simulink model "nmsRR"  (R2021a)
settings: Solver=ode15s  StartTime=0.0  StopTime=t  MaxStep=1e-2  RelTol=1e-2
StartFcn:
  | tic
StopFcn:
  | toc
  | 
  | 
  | %if GimbalLockFlag
  |  % fprintf(2, 'Almost reached Gimbal Lock of IMU. Simulation stopped.\n')
  | %end
  | 
  | %fprintf('Elapsed time: %4.2f sec (%4.2f%% realtime)\n', a, tout(end)/a*100)
undefined symbols (not defined in the file): Balance02, Balance13, BalanceTrunk, BasisStim, CompensateSwing, CompliantLeg, FlexAnkle, Ground, ICs, init_des_left, init_des_right, init_l_left, init_l_right, init_q_del, init_sensor_body, init_sensor_world, init_v_left, init_v_right, LateralControl, mParams, PreventKneeOverextension, StepDur, Target02, Target13, theta0, X, Y, Z
libraries: simulink_extras x133, nesl_utility x105, sm_lib x88, simulink x72, robotcorelib x5, dspinverses x5, dspswit3 x2, vrlib x2, robotmaniplib x1
(part 6 of 8)

== system nmsRR/Spinal Layer/Stretch Reflex for Swing Leg Control/LPF 11x0.0025s ==
  in : Inport
  Demux2 : Demux  Outputs=11
  Mux2 : Mux  Inputs=11
  Transfer Fcn (with initial outputs)1 : simulink_extras/Additional Linear/Transfer Fcn (with initial outputs)  N=[1]  D="[0.0025  1]"  Y0=init_des_left(1)  U0=init_des_left(1)
  Transfer Fcn (with initial outputs)10 : simulink_extras/Additional Linear/Transfer Fcn (with initial outputs)  N=[1]  D="[0.0025  1]"  Y0=init_des_left(10)  U0=init_des_left(10)
  Transfer Fcn (with initial outputs)11 : simulink_extras/Additional Linear/Transfer Fcn (with initial outputs)  N=[1]  D="[0.0025  1]"  Y0=init_des_left(11)  U0=init_des_left(11)
  Transfer Fcn (with initial outputs)2 : simulink_extras/Additional Linear/Transfer Fcn (with initial outputs)  N=[1]  D="[0.0025  1]"  Y0=init_des_left(2)  U0=init_des_left(2)
  Transfer Fcn (with initial outputs)3 : simulink_extras/Additional Linear/Transfer Fcn (with initial outputs)  N=[1]  D="[0.0025  1]"  Y0=init_des_left(3)  U0=init_des_left(3)
  Transfer Fcn (with initial outputs)4 : simulink_extras/Additional Linear/Transfer Fcn (with initial outputs)  N=[1]  D="[0.0025  1]"  Y0=init_des_left(4)  U0=init_des_left(4)
  Transfer Fcn (with initial outputs)5 : simulink_extras/Additional Linear/Transfer Fcn (with initial outputs)  N=[1]  D="[0.0025  1]"  Y0=init_des_left(5)  U0=init_des_left(5)
  Transfer Fcn (with initial outputs)6 : simulink_extras/Additional Linear/Transfer Fcn (with initial outputs)  N=[1]  D="[0.0025  1]"  Y0=init_des_left(6)  U0=init_des_left(6)
  Transfer Fcn (with initial outputs)7 : simulink_extras/Additional Linear/Transfer Fcn (with initial outputs)  N=[1]  D="[0.0025  1]"  Y0=init_des_left(7)  U0=init_des_left(7)
  Transfer Fcn (with initial outputs)8 : simulink_extras/Additional Linear/Transfer Fcn (with initial outputs)  N=[1]  D="[0.0025  1]"  Y0=init_des_left(8)  U0=init_des_left(8)
  Transfer Fcn (with initial outputs)9 : simulink_extras/Additional Linear/Transfer Fcn (with initial outputs)  N=[1]  D="[0.0025  1]"  Y0=init_des_left(9)  U0=init_des_left(9)
  lambda : Outport
  wires:
  Mux2/1 -> lambda/1
  Demux2/1 -> Transfer Fcn (with initial outputs)1/1
  Transfer Fcn (with initial outputs)6/1 -> Mux2/6
  Transfer Fcn (with initial outputs)3/1 -> Mux2/3
  Transfer Fcn (with initial outputs)10/1 -> Mux2/10
  Demux2/2 -> Transfer Fcn (with initial outputs)2/1
  Transfer Fcn (with initial outputs)7/1 -> Mux2/7
  Demux2/10 -> Transfer Fcn (with initial outputs)10/1
  Transfer Fcn (with initial outputs)9/1 -> Mux2/9
  Demux2/9 -> Transfer Fcn (with initial outputs)9/1
  in/1 -> Demux2/1
  Transfer Fcn (with initial outputs)4/1 -> Mux2/4
  Transfer Fcn (with initial outputs)8/1 -> Mux2/8
  Transfer Fcn (with initial outputs)5/1 -> Mux2/5
  Transfer Fcn (with initial outputs)11/1 -> Mux2/11
  Demux2/11 -> Transfer Fcn (with initial outputs)11/1
  Demux2/7 -> Transfer Fcn (with initial outputs)7/1
  Demux2/3 -> Transfer Fcn (with initial outputs)3/1
  Demux2/6 -> Transfer Fcn (with initial outputs)6/1
  Transfer Fcn (with initial outputs)1/1 -> Mux2/1
  Demux2/5 -> Transfer Fcn (with initial outputs)5/1
  Transfer Fcn (with initial outputs)2/1 -> Mux2/2
  Demux2/4 -> Transfer Fcn (with initial outputs)4/1
  Demux2/8 -> Transfer Fcn (with initial outputs)8/1

== system nmsRR/Spinal Layer/Stretch Reflex for Swing Leg Control/LPF 11x0.0025s1 ==
  in : Inport
  Demux2 : Demux  Outputs=11
  Mux2 : Mux  Inputs=11
  Transfer Fcn (with initial outputs)1 : simulink_extras/Additional Linear/Transfer Fcn (with initial outputs)  N=[1]  D="[0.0025  1]"  Y0=init_l_left(1)  U0=init_l_left(1)
  Transfer Fcn (with initial outputs)10 : simulink_extras/Additional Linear/Transfer Fcn (with initial outputs)  N=[1]  D="[0.0025  1]"  Y0=init_l_left(10)  U0=init_l_left(10)
  Transfer Fcn (with initial outputs)11 : simulink_extras/Additional Linear/Transfer Fcn (with initial outputs)  N=[1]  D="[0.0025  1]"  Y0=init_l_left(11)  U0=init_l_left(11)
  Transfer Fcn (with initial outputs)2 : simulink_extras/Additional Linear/Transfer Fcn (with initial outputs)  N=[1]  D="[0.0025  1]"  Y0=init_l_left(2)  U0=init_l_left(2)
  Transfer Fcn (with initial outputs)3 : simulink_extras/Additional Linear/Transfer Fcn (with initial outputs)  N=[1]  D="[0.0025  1]"  Y0=init_l_left(3)  U0=init_l_left(3)
  Transfer Fcn (with initial outputs)4 : simulink_extras/Additional Linear/Transfer Fcn (with initial outputs)  N=[1]  D="[0.0025  1]"  Y0=init_l_left(4)  U0=init_l_left(4)
  Transfer Fcn (with initial outputs)5 : simulink_extras/Additional Linear/Transfer Fcn (with initial outputs)  N=[1]  D="[0.0025  1]"  Y0=init_l_left(5)  U0=init_l_left(5)
  Transfer Fcn (with initial outputs)6 : simulink_extras/Additional Linear/Transfer Fcn (with initial outputs)  N=[1]  D="[0.0025  1]"  Y0=init_l_left(6)  U0=init_l_left(6)
  Transfer Fcn (with initial outputs)7 : simulink_extras/Additional Linear/Transfer Fcn (with initial outputs)  N=[1]  D="[0.0025  1]"  Y0=init_l_left(7)  U0=init_l_left(7)
  Transfer Fcn (with initial outputs)8 : simulink_extras/Additional Linear/Transfer Fcn (with initial outputs)  N=[1]  D="[0.0025  1]"  Y0=init_l_left(8)  U0=init_l_left(8)
  Transfer Fcn (with initial outputs)9 : simulink_extras/Additional Linear/Transfer Fcn (with initial outputs)  N=[1]  D="[0.0025  1]"  Y0=init_l_left(9)  U0=init_l_left(9)
  l : Outport
  wires:
  Mux2/1 -> l/1
  Demux2/1 -> Transfer Fcn (with initial outputs)1/1
  Transfer Fcn (with initial outputs)6/1 -> Mux2/6
  Transfer Fcn (with initial outputs)3/1 -> Mux2/3
  Transfer Fcn (with initial outputs)10/1 -> Mux2/10
  Demux2/2 -> Transfer Fcn (with initial outputs)2/1
  Transfer Fcn (with initial outputs)7/1 -> Mux2/7
  Demux2/10 -> Transfer Fcn (with initial outputs)10/1
  Transfer Fcn (with initial outputs)9/1 -> Mux2/9
  Demux2/9 -> Transfer Fcn (with initial outputs)9/1
  in/1 -> Demux2/1
  Transfer Fcn (with initial outputs)4/1 -> Mux2/4
  Transfer Fcn (with initial outputs)8/1 -> Mux2/8
  Transfer Fcn (with initial outputs)5/1 -> Mux2/5
  Transfer Fcn (with initial outputs)11/1 -> Mux2/11
  Demux2/11 -> Transfer Fcn (with initial outputs)11/1
  Demux2/7 -> Transfer Fcn (with initial outputs)7/1
  Demux2/3 -> Transfer Fcn (with initial outputs)3/1
  Demux2/6 -> Transfer Fcn (with initial outputs)6/1
  Transfer Fcn (with initial outputs)1/1 -> Mux2/1
  Demux2/5 -> Transfer Fcn (with initial outputs)5/1
  Transfer Fcn (with initial outputs)2/1 -> Mux2/2
  Demux2/4 -> Transfer Fcn (with initial outputs)4/1
  Demux2/8 -> Transfer Fcn (with initial outputs)8/1

== system nmsRR/Spinal Layer/Stretch Reflex for Swing Leg Control/LPF 11x0.0025s2 ==
  in : Inport
  Demux2 : Demux  Outputs=11
  Mux2 : Mux  Inputs=11
  Transfer Fcn (with initial outputs)1 : simulink_extras/Additional Linear/Transfer Fcn (with initial outputs)  N=[1]  D="[0.0025  1]"  Y0=init_v_left(1)  U0=init_v_left(1)
  Transfer Fcn (with initial outputs)10 : simulink_extras/Additional Linear/Transfer Fcn (with initial outputs)  N=[1]  D="[0.0025  1]"  Y0=init_v_left(10)  U0=init_v_left(10)
  Transfer Fcn (with initial outputs)11 : simulink_extras/Additional Linear/Transfer Fcn (with initial outputs)  N=[1]  D="[0.0025  1]"  Y0=init_v_left(11)  U0=init_v_left(11)
  Transfer Fcn (with initial outputs)2 : simulink_extras/Additional Linear/Transfer Fcn (with initial outputs)  N=[1]  D="[0.0025  1]"  Y0=init_v_left(2)  U0=init_v_left(2)
  Transfer Fcn (with initial outputs)3 : simulink_extras/Additional Linear/Transfer Fcn (with initial outputs)  N=[1]  D="[0.0025  1]"  Y0=init_v_left(3)  U0=init_v_left(3)
  Transfer Fcn (with initial outputs)4 : simulink_extras/Additional Linear/Transfer Fcn (with initial outputs)  N=[1]  D="[0.0025  1]"  Y0=init_v_left(4)  U0=init_v_left(4)
  Transfer Fcn (with initial outputs)5 : simulink_extras/Additional Linear/Transfer Fcn (with initial outputs)  N=[1]  D="[0.0025  1]"  Y0=init_v_left(5)  U0=init_v_left(5)
  Transfer Fcn (with initial outputs)6 : simulink_extras/Additional Linear/Transfer Fcn (with initial outputs)  N=[1]  D="[0.0025  1]"  Y0=init_v_left(6)  U0=init_v_left(6)
  Transfer Fcn (with initial outputs)7 : simulink_extras/Additional Linear/Transfer Fcn (with initial outputs)  N=[1]  D="[0.0025  1]"  Y0=init_v_left(7)  U0=init_v_left(7)
  Transfer Fcn (with initial outputs)8 : simulink_extras/Additional Linear/Transfer Fcn (with initial outputs)  N=[1]  D="[0.0025  1]"  Y0=init_v_left(8)  U0=init_v_left(8)
  Transfer Fcn (with initial outputs)9 : simulink_extras/Additional Linear/Transfer Fcn (with initial outputs)  N=[1]  D="[0.0025  1]"  Y0=init_v_left(9)  U0=init_v_left(9)
  v : Outport
  wires:
  Mux2/1 -> v/1
  Demux2/1 -> Transfer Fcn (with initial outputs)1/1
  Transfer Fcn (with initial outputs)6/1 -> Mux2/6
  Transfer Fcn (with initial outputs)3/1 -> Mux2/3
  Transfer Fcn (with initial outputs)10/1 -> Mux2/10
  Demux2/2 -> Transfer Fcn (with initial outputs)2/1
  Transfer Fcn (with initial outputs)7/1 -> Mux2/7
  Demux2/10 -> Transfer Fcn (with initial outputs)10/1
  Transfer Fcn (with initial outputs)9/1 -> Mux2/9
  Demux2/9 -> Transfer Fcn (with initial outputs)9/1
  in/1 -> Demux2/1
  Transfer Fcn (with initial outputs)4/1 -> Mux2/4
  Transfer Fcn (with initial outputs)8/1 -> Mux2/8
  Transfer Fcn (with initial outputs)5/1 -> Mux2/5
  Transfer Fcn (with initial outputs)11/1 -> Mux2/11
  Demux2/11 -> Transfer Fcn (with initial outputs)11/1
  Demux2/7 -> Transfer Fcn (with initial outputs)7/1
  Demux2/3 -> Transfer Fcn (with initial outputs)3/1
  Demux2/6 -> Transfer Fcn (with initial outputs)6/1
  Transfer Fcn (with initial outputs)1/1 -> Mux2/1
  Demux2/5 -> Transfer Fcn (with initial outputs)5/1
  Transfer Fcn (with initial outputs)2/1 -> Mux2/2
  Demux2/4 -> Transfer Fcn (with initial outputs)4/1
  Demux2/8 -> Transfer Fcn (with initial outputs)8/1

== system nmsRR/Spinal Layer/Stretch Reflex for Swing Leg Control/LPF 11x0.0025s3 ==
  in : Inport
  Demux2 : Demux  Outputs=11
  Mux2 : Mux  Inputs=11
  Transfer Fcn (with initial outputs)1 : simulink_extras/Additional Linear/Transfer Fcn (with initial outputs)  N=[1]  D="[0.0025  1]"  Y0=init_des_right(1)  U0=init_des_right(1)
  Transfer Fcn (with initial outputs)10 : simulink_extras/Additional Linear/Transfer Fcn (with initial outputs)  N=[1]  D="[0.0025  1]"  Y0=init_des_right(10)  U0=init_des_right(10)
  Transfer Fcn (with initial outputs)11 : simulink_extras/Additional Linear/Transfer Fcn (with initial outputs)  N=[1]  D="[0.0025  1]"  Y0=init_des_right(11)  U0=init_des_right(11)
  Transfer Fcn (with initial outputs)2 : simulink_extras/Additional Linear/Transfer Fcn (with initial outputs)  N=[1]  D="[0.0025  1]"  Y0=init_des_right(2)  U0=init_des_right(2)
  Transfer Fcn (with initial outputs)3 : simulink_extras/Additional Linear/Transfer Fcn (with initial outputs)  N=[1]  D="[0.0025  1]"  Y0=init_des_right(3)  U0=init_des_right(3)
  Transfer Fcn (with initial outputs)4 : simulink_extras/Additional Linear/Transfer Fcn (with initial outputs)  N=[1]  D="[0.0025  1]"  Y0=init_des_right(4)  U0=init_des_right(4)
  Transfer Fcn (with initial outputs)5 : simulink_extras/Additional Linear/Transfer Fcn (with initial outputs)  N=[1]  D="[0.0025  1]"  Y0=init_des_right(5)  U0=init_des_right(5)
  Transfer Fcn (with initial outputs)6 : simulink_extras/Additional Linear/Transfer Fcn (with initial outputs)  N=[1]  D="[0.0025  1]"  Y0=init_des_right(6)  U0=init_des_right(6)
  Transfer Fcn (with initial outputs)7 : simulink_extras/Additional Linear/Transfer Fcn (with initial outputs)  N=[1]  D="[0.0025  1]"  Y0=init_des_right(7)  U0=init_des_right(7)
  Transfer Fcn (with initial outputs)8 : simulink_extras/Additional Linear/Transfer Fcn (with initial outputs)  N=[1]  D="[0.0025  1]"  Y0=init_des_right(8)  U0=init_des_right(8)
  Transfer Fcn (with initial outputs)9 : simulink_extras/Additional Linear/Transfer Fcn (with initial outputs)  N=[1]  D="[0.0025  1]"  Y0=init_des_right(9)  U0=init_des_right(9)
  lambda : Outport
  wires:
  Mux2/1 -> lambda/1
  Demux2/1 -> Transfer Fcn (with initial outputs)1/1
  Transfer Fcn (with initial outputs)6/1 -> Mux2/6
  Transfer Fcn (with initial outputs)3/1 -> Mux2/3
  Transfer Fcn (with initial outputs)10/1 -> Mux2/10
  Demux2/2 -> Transfer Fcn (with initial outputs)2/1
  Transfer Fcn (with initial outputs)7/1 -> Mux2/7
  Demux2/10 -> Transfer Fcn (with initial outputs)10/1
  Transfer Fcn (with initial outputs)9/1 -> Mux2/9
  Demux2/9 -> Transfer Fcn (with initial outputs)9/1
  in/1 -> Demux2/1
  Transfer Fcn (with initial outputs)4/1 -> Mux2/4
  Transfer Fcn (with initial outputs)8/1 -> Mux2/8
  Transfer Fcn (with initial outputs)5/1 -> Mux2/5
  Transfer Fcn (with initial outputs)11/1 -> Mux2/11
  Demux2/11 -> Transfer Fcn (with initial outputs)11/1
  Demux2/7 -> Transfer Fcn (with initial outputs)7/1
  Demux2/3 -> Transfer Fcn (with initial outputs)3/1
  Demux2/6 -> Transfer Fcn (with initial outputs)6/1
  Transfer Fcn (with initial outputs)1/1 -> Mux2/1
  Demux2/5 -> Transfer Fcn (with initial outputs)5/1
  Transfer Fcn (with initial outputs)2/1 -> Mux2/2
  Demux2/4 -> Transfer Fcn (with initial outputs)4/1
  Demux2/8 -> Transfer Fcn (with initial outputs)8/1

== system nmsRR/Spinal Layer/Stretch Reflex for Swing Leg Control/LPF 11x0.0025s4 ==
  in : Inport
  Demux2 : Demux  Outputs=11
  Mux2 : Mux  Inputs=11
  Transfer Fcn (with initial outputs)1 : simulink_extras/Additional Linear/Transfer Fcn (with initial outputs)  N=[1]  D="[0.0025  1]"  Y0=init_l_right(1)  U0=init_l_right(1)
  Transfer Fcn (with initial outputs)10 : simulink_extras/Additional Linear/Transfer Fcn (with initial outputs)  N=[1]  D="[0.0025  1]"  Y0=init_l_right(10)  U0=init_l_right(10)
  Transfer Fcn (with initial outputs)11 : simulink_extras/Additional Linear/Transfer Fcn (with initial outputs)  N=[1]  D="[0.0025  1]"  Y0=init_l_right(11)  U0=init_l_right(11)
  Transfer Fcn (with initial outputs)2 : simulink_extras/Additional Linear/Transfer Fcn (with initial outputs)  N=[1]  D="[0.0025  1]"  Y0=init_l_right(2)  U0=init_l_right(2)
  Transfer Fcn (with initial outputs)3 : simulink_extras/Additional Linear/Transfer Fcn (with initial outputs)  N=[1]  D="[0.0025  1]"  Y0=init_l_right(3)  U0=init_l_right(3)
  Transfer Fcn (with initial outputs)4 : simulink_extras/Additional Linear/Transfer Fcn (with initial outputs)  N=[1]  D="[0.0025  1]"  Y0=init_l_right(4)  U0=init_l_right(4)
  Transfer Fcn (with initial outputs)5 : simulink_extras/Additional Linear/Transfer Fcn (with initial outputs)  N=[1]  D="[0.0025  1]"  Y0=init_l_right(5)  U0=init_l_right(5)
  Transfer Fcn (with initial outputs)6 : simulink_extras/Additional Linear/Transfer Fcn (with initial outputs)  N=[1]  D="[0.0025  1]"  Y0=init_l_right(6)  U0=init_l_right(6)
  Transfer Fcn (with initial outputs)7 : simulink_extras/Additional Linear/Transfer Fcn (with initial outputs)  N=[1]  D="[0.0025  1]"  Y0=init_l_right(7)  U0=init_l_right(7)
  Transfer Fcn (with initial outputs)8 : simulink_extras/Additional Linear/Transfer Fcn (with initial outputs)  N=[1]  D="[0.0025  1]"  Y0=init_l_right(8)  U0=init_l_right(8)
  Transfer Fcn (with initial outputs)9 : simulink_extras/Additional Linear/Transfer Fcn (with initial outputs)  N=[1]  D="[0.0025  1]"  Y0=init_l_right(9)  U0=init_l_right(9)
  l : Outport
  wires:
  Mux2/1 -> l/1
  Demux2/1 -> Transfer Fcn (with initial outputs)1/1
  Transfer Fcn (with initial outputs)6/1 -> Mux2/6
  Transfer Fcn (with initial outputs)3/1 -> Mux2/3
  Transfer Fcn (with initial outputs)10/1 -> Mux2/10
  Demux2/2 -> Transfer Fcn (with initial outputs)2/1
  Transfer Fcn (with initial outputs)7/1 -> Mux2/7
  Demux2/10 -> Transfer Fcn (with initial outputs)10/1
  Transfer Fcn (with initial outputs)9/1 -> Mux2/9
  Demux2/9 -> Transfer Fcn (with initial outputs)9/1
  in/1 -> Demux2/1
  Transfer Fcn (with initial outputs)4/1 -> Mux2/4
  Transfer Fcn (with initial outputs)8/1 -> Mux2/8
  Transfer Fcn (with initial outputs)5/1 -> Mux2/5
  Transfer Fcn (with initial outputs)11/1 -> Mux2/11
  Demux2/11 -> Transfer Fcn (with initial outputs)11/1
  Demux2/7 -> Transfer Fcn (with initial outputs)7/1
  Demux2/3 -> Transfer Fcn (with initial outputs)3/1
  Demux2/6 -> Transfer Fcn (with initial outputs)6/1
  Transfer Fcn (with initial outputs)1/1 -> Mux2/1
  Demux2/5 -> Transfer Fcn (with initial outputs)5/1
  Transfer Fcn (with initial outputs)2/1 -> Mux2/2
  Demux2/4 -> Transfer Fcn (with initial outputs)4/1
  Demux2/8 -> Transfer Fcn (with initial outputs)8/1

== system nmsRR/Spinal Layer/Stretch Reflex for Swing Leg Control/LPF 11x0.0025s5 ==
  in : Inport
  Demux2 : Demux  Outputs=11
  Mux2 : Mux  Inputs=11
  Transfer Fcn (with initial outputs){1..11} (11 alike) : simulink_extras/Additional Linear/Transfer Fcn (with initial outputs)  N=[ 1 0]  D="[0.0025  1]"  Y0=0  U0=0
  lambda dot : Outport
  wires:
  Mux2/1 -> lambda dot/1
  Demux2/1 -> Transfer Fcn (with initial outputs)1/1
  Transfer Fcn (with initial outputs)6/1 -> Mux2/6
  Transfer Fcn (with initial outputs)3/1 -> Mux2/3
  Transfer Fcn (with initial outputs)10/1 -> Mux2/10
  Demux2/2 -> Transfer Fcn (with initial outputs)2/1
  Transfer Fcn (with initial outputs)7/1 -> Mux2/7
  Demux2/10 -> Transfer Fcn (with initial outputs)10/1
  Transfer Fcn (with initial outputs)9/1 -> Mux2/9
  Demux2/9 -> Transfer Fcn (with initial outputs)9/1
  in/1 -> Demux2/1
  Transfer Fcn (with initial outputs)4/1 -> Mux2/4
  Transfer Fcn (with initial outputs)8/1 -> Mux2/8
  Transfer Fcn (with initial outputs)5/1 -> Mux2/5
  Transfer Fcn (with initial outputs)11/1 -> Mux2/11
  Demux2/11 -> Transfer Fcn (with initial outputs)11/1
  Demux2/7 -> Transfer Fcn (with initial outputs)7/1
  Demux2/3 -> Transfer Fcn (with initial outputs)3/1
  Demux2/6 -> Transfer Fcn (with initial outputs)6/1
  Transfer Fcn (with initial outputs)1/1 -> Mux2/1
  Demux2/5 -> Transfer Fcn (with initial outputs)5/1
  Transfer Fcn (with initial outputs)2/1 -> Mux2/2
  Demux2/4 -> Transfer Fcn (with initial outputs)4/1
  Demux2/8 -> Transfer Fcn (with initial outputs)8/1

== system nmsRR/Spinal Layer/Stretch Reflex for Swing Leg Control/LPF 11x0.0025s6 ==
  in : Inport
  Demux2 : Demux  Outputs=11
  Mux2 : Mux  Inputs=11
  Transfer Fcn (with initial outputs)1 : simulink_extras/Additional Linear/Transfer Fcn (with initial outputs)  N=[1]  D="[0.0025  1]"  Y0=init_v_right(1)  U0=init_v_right(1)
  Transfer Fcn (with initial outputs)10 : simulink_extras/Additional Linear/Transfer Fcn (with initial outputs)  N=[1]  D="[0.0025  1]"  Y0=init_v_right(10)  U0=init_v_right(10)
  Transfer Fcn (with initial outputs)11 : simulink_extras/Additional Linear/Transfer Fcn (with initial outputs)  N=[1]  D="[0.0025  1]"  Y0=init_v_right(11)  U0=init_v_right(11)
  Transfer Fcn (with initial outputs)2 : simulink_extras/Additional Linear/Transfer Fcn (with initial outputs)  N=[1]  D="[0.0025  1]"  Y0=init_v_right(2)  U0=init_v_right(2)
  Transfer Fcn (with initial outputs)3 : simulink_extras/Additional Linear/Transfer Fcn (with initial outputs)  N=[1]  D="[0.0025  1]"  Y0=init_v_right(3)  U0=init_v_right(3)
  Transfer Fcn (with initial outputs)4 : simulink_extras/Additional Linear/Transfer Fcn (with initial outputs)  N=[1]  D="[0.0025  1]"  Y0=init_v_right(4)  U0=init_v_right(4)
  Transfer Fcn (with initial outputs)5 : simulink_extras/Additional Linear/Transfer Fcn (with initial outputs)  N=[1]  D="[0.0025  1]"  Y0=init_v_right(5)  U0=init_v_right(5)
  Transfer Fcn (with initial outputs)6 : simulink_extras/Additional Linear/Transfer Fcn (with initial outputs)  N=[1]  D="[0.0025  1]"  Y0=init_v_right(6)  U0=init_v_right(6)
  Transfer Fcn (with initial outputs)7 : simulink_extras/Additional Linear/Transfer Fcn (with initial outputs)  N=[1]  D="[0.0025  1]"  Y0=init_v_right(7)  U0=init_v_right(7)
  Transfer Fcn (with initial outputs)8 : simulink_extras/Additional Linear/Transfer Fcn (with initial outputs)  N=[1]  D="[0.0025  1]"  Y0=init_v_right(8)  U0=init_v_right(8)
  Transfer Fcn (with initial outputs)9 : simulink_extras/Additional Linear/Transfer Fcn (with initial outputs)  N=[1]  D="[0.0025  1]"  Y0=init_v_right(9)  U0=init_v_right(9)
  v : Outport
  wires:
  Mux2/1 -> v/1
  Demux2/1 -> Transfer Fcn (with initial outputs)1/1
  Transfer Fcn (with initial outputs)6/1 -> Mux2/6
  Transfer Fcn (with initial outputs)3/1 -> Mux2/3
  Transfer Fcn (with initial outputs)10/1 -> Mux2/10
  Demux2/2 -> Transfer Fcn (with initial outputs)2/1
  Transfer Fcn (with initial outputs)7/1 -> Mux2/7
  Demux2/10 -> Transfer Fcn (with initial outputs)10/1
  Transfer Fcn (with initial outputs)9/1 -> Mux2/9
  Demux2/9 -> Transfer Fcn (with initial outputs)9/1
  in/1 -> Demux2/1
  Transfer Fcn (with initial outputs)4/1 -> Mux2/4
  Transfer Fcn (with initial outputs)8/1 -> Mux2/8
  Transfer Fcn (with initial outputs)5/1 -> Mux2/5
  Transfer Fcn (with initial outputs)11/1 -> Mux2/11
  Demux2/11 -> Transfer Fcn (with initial outputs)11/1
  Demux2/7 -> Transfer Fcn (with initial outputs)7/1
  Demux2/3 -> Transfer Fcn (with initial outputs)3/1
  Demux2/6 -> Transfer Fcn (with initial outputs)6/1
  Transfer Fcn (with initial outputs)1/1 -> Mux2/1
  Demux2/5 -> Transfer Fcn (with initial outputs)5/1
  Transfer Fcn (with initial outputs)2/1 -> Mux2/2
  Demux2/4 -> Transfer Fcn (with initial outputs)4/1
  Demux2/8 -> Transfer Fcn (with initial outputs)8/1

== system nmsRR/Spinal Layer/Stretch Reflex for Swing Leg Control/LPF 11x0.0025s7 ==
  in : Inport
  Demux2 : Demux  Outputs=11
  Mux2 : Mux  Inputs=11
  Transfer Fcn (with initial outputs){1..11} (11 alike) : simulink_extras/Additional Linear/Transfer Fcn (with initial outputs)  N=[ 1 0]  D="[0.0025  1]"  Y0=0  U0=0
  lambda dot : Outport
  wires:
  Mux2/1 -> lambda dot/1
  Demux2/1 -> Transfer Fcn (with initial outputs)1/1
  Transfer Fcn (with initial outputs)6/1 -> Mux2/6
  Transfer Fcn (with initial outputs)3/1 -> Mux2/3
  Transfer Fcn (with initial outputs)10/1 -> Mux2/10
  Demux2/2 -> Transfer Fcn (with initial outputs)2/1
  Transfer Fcn (with initial outputs)7/1 -> Mux2/7
  Demux2/10 -> Transfer Fcn (with initial outputs)10/1
  Transfer Fcn (with initial outputs)9/1 -> Mux2/9
  Demux2/9 -> Transfer Fcn (with initial outputs)9/1
  in/1 -> Demux2/1
  Transfer Fcn (with initial outputs)4/1 -> Mux2/4
  Transfer Fcn (with initial outputs)8/1 -> Mux2/8
  Transfer Fcn (with initial outputs)5/1 -> Mux2/5
  Transfer Fcn (with initial outputs)11/1 -> Mux2/11
  Demux2/11 -> Transfer Fcn (with initial outputs)11/1
  Demux2/7 -> Transfer Fcn (with initial outputs)7/1
  Demux2/3 -> Transfer Fcn (with initial outputs)3/1
  Demux2/6 -> Transfer Fcn (with initial outputs)6/1
  Transfer Fcn (with initial outputs)1/1 -> Mux2/1
  Demux2/5 -> Transfer Fcn (with initial outputs)5/1
  Transfer Fcn (with initial outputs)2/1 -> Mux2/2
  Demux2/4 -> Transfer Fcn (with initial outputs)4/1
  Demux2/8 -> Transfer Fcn (with initial outputs)8/1

== system nmsRR/Spinal Layer/Stretch Reflex for Swing Leg Control/Stretch Reflex Left ==
  lambda : Inport
  lambda_dot : Inport  Port=2
  l_ce : Inport  Port=3
  v_ce : Inport  Port=4
  Add2 : Sum  Inputs=-+
  Add3 : Sum  Inputs=-+
  Add7 : Sum
  Gain10 : Gain  Gain=0.03
  Gain9 : Gain  Gain=mParams.muscles.K
  STIM : Outport  VectorParamsAs1DForOutWhenUnconnected=off
  wires:
  lambda/1 -> Add2/1
  Add7/1 -> STIM/1
  Gain9/1 -> Add7/1
  Gain10/1 -> Add7/2
  Add3/1 -> Gain10/1
  Add2/1 -> Gain9/1
  v_ce/1 -> Add3/2
  l_ce/1 -> Add2/2
  lambda_dot/1 -> Add3/1

== system nmsRR/Spinal Layer/Stretch Reflex for Swing Leg Control/Stretch Reflex Right ==
  lambda : Inport
  lambda_dot : Inport  Port=2
  l_ce : Inport  Port=3
  v_ce : Inport  Port=4
  Add2 : Sum  Inputs=-+
  Add3 : Sum  Inputs=-+
  Add7 : Sum
  Gain1 : Gain  Commented=on  Gain=[ 0.03 0.03 0.03 0.03 0.03 0.03 0.03 0.03 0.1 0.1 0.1]
  Gain10 : Gain  Gain=0.03
  Gain9 : Gain  Gain=mParams.muscles.K
  STIM : Outport  VectorParamsAs1DForOutWhenUnconnected=off
  wires:
  lambda/1 -> Add2/1
  Add7/1 -> STIM/1
  Gain9/1 -> Add7/1
  Gain10/1 -> Add7/2
  Add3/1 -> Gain10/1
  Add2/1 -> Gain9/1
  v_ce/1 -> Add3/2
  l_ce/1 -> Add2/2
  lambda_dot/1 -> Add3/1

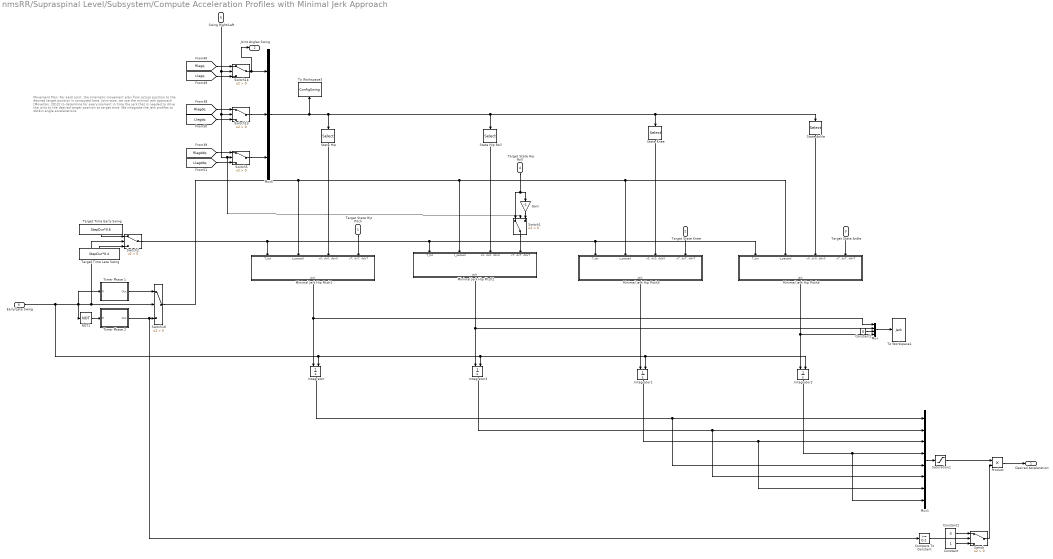
== system nmsRR/Supraspinal Level/Subsystem/Compute Acceleration Profiles with Minimal Jerk Approach ==
  note: Movement Plan: For each joint, the kinematic movement plan from actual position to the desired target position is computed here. Joint-wise, we use the mininal jerk approach [Movellan, 2012] to determine for every moment in time the jerk that is needed to drive the joint to the desired target position at target time. We integrate the jerk profiles to obtain angle accelerations.
  Target State Hip Pitch : Inport
  Target State Knee : Inport  Port=2
  Target State Ankle : Inport  Port=3
  Target State Hip Roll : Inport  Port=4
  Swing Right/Left : Inport  Port=5
  Early/Late Swing : Inport  Port=6
  " Timer Phase 1" : Subsystem
  " Timer Phase 2" : Subsystem
  Compare To Constant : simulink/Logic and Bit Operations/Compare To Constant  relop=>=  const=0.2  OutDataTypeStr=boolean  ZeroCross=off
  Constant : Constant
  Constant1 : Constant  Value=0
  Constant2 : Constant  Value=0
  Gain : Gain  Gain=-1
  Integrator{,1..3} (4 alike) : Integrator  ExternalReset=either  ZeroCross=off
  Minimal jerk Hip Pitch1 : Subsystem
  Minimal jerk Hip Pitch2 : Subsystem
  Minimal jerk Hip Pitch3 : Subsystem
  Minimal jerk Hip Pitch4 : Subsystem
  Mux : Mux
  Mux1 : Mux  Inputs=8
  Mux5 : Mux  Inputs=3
  NOT1 : Logic  Operator=NOT  AllPortsSameDT=off  OutDataTypeStr=boolean
  Product : Product
  Saturation1 : Saturate  UpperLimit=2000  LowerLimit=-2000  ZeroCross=off
  State Ankle : Selector  InputPortWidth=12  IndexOptions=Index vector (dialog)  Indices=[4 8 12]  OutputSizes=1
  State Hip : Selector  InputPortWidth=12  IndexOptions=Index vector (dialog)  Indices=[1 5 9]  OutputSizes=1
  State Hip Roll : Selector  InputPortWidth=12  IndexOptions=Index vector (dialog)  Indices=[2 6 10 ]  OutputSizes=1
  State Knee : Selector  InputPortWidth=12  IndexOptions=Index vector (dialog)  Indices=[3 7 11 ]  OutputSizes=1
  Switch{,1..2,5,13..14,16} (7 alike) : Switch  Criteria=u2 > Threshold  ZeroCross=off
  Target Time Early Swing : Constant  Value=StepDur*0.6
  Target Time Late Swing : Constant  Value=StepDur*0.4
  To Workspace1 : ToWorkspace  VariableName=Jerk  SampleTime=-1
      settings: Save2DSignal=2-D array (concatenate along first dimension)
  To Workspace3 : ToWorkspace  VariableName=ConfigSwing  SampleTime=-1
      settings: Save2DSignal=2-D array (concatenate along first dimension)
  "Desired Acceleration " : Outport
  Joint Angles Swing : Outport  Port=2
  wires:
  State Hip/1 -> Minimal jerk Hip Pitch1/3("x0, dx0, ddx0")
  NOT1/1 -> " Timer Phase 2"/1(R)
  Mux1/1 -> Saturation1/1
  Switch2/1 -> Minimal jerk Hip Pitch1/1(T_tot), Minimal jerk Hip Pitch2/1(T_tot), Minimal jerk Hip Pitch4/1(T_tot), Minimal jerk Hip Pitch3/1(T_tot)
  [Llegddq] -> Switch5/3
  [Rlegq] -> Switch14/1
  [Llegdq] -> Switch13/3
  Target State Hip Pitch/1 -> Minimal jerk Hip Pitch1/4("xT, dxT, ddxT")
  Target State Knee/1 -> Minimal jerk Hip Pitch3/4("xT, dxT, ddxT")
  [Rlegddq] -> Switch5/1
  Integrator1/1 -> Mux1/3, Mux1/7
  Switch5/1 -> Mux5/3
  [Llegq] -> Switch14/3
  State Knee/1 -> Minimal jerk Hip Pitch3/3("x0, dx0, ddx0")
  Target State Ankle/1 -> Minimal jerk Hip Pitch4/4("xT, dxT, ddxT")
  Integrator/1 -> Mux1/1, Mux1/5
  Switch14/1 -> Joint Angles Swing/1, Mux5/1
  Integrator2/1 -> Mux1/4, Mux1/8
  State Ankle/1 -> Minimal jerk Hip Pitch4/3("x0, dx0, ddx0")
  Switch13/1 -> Mux5/2
  [Rlegdq] -> Switch13/1
  Early/Late Swing/1 -> Switch2/2, Switch16/2, NOT1/1, " Timer Phase 1"/1(R), Integrator3/2, Integrator2/2, Integrator1/2, Integrator/2
  Swing Right/Left/1 -> Switch14/2, Switch13/2, Switch1/2, Switch5/2
  Switch16/1 -> Minimal jerk Hip Pitch1/2(t_passed), Minimal jerk Hip Pitch2/2(t_passed), Minimal jerk Hip Pitch4/2(t_passed), Minimal jerk Hip Pitch3/2(t_passed)
  State Hip Roll/1 -> Minimal jerk Hip Pitch2/3("x0, dx0, ddx0")
  Integrator3/1 -> Mux1/2, Mux1/6
  Switch1/1 -> Minimal jerk Hip Pitch2/4("xT, dxT, ddxT")
  Target State Hip Roll/1 -> Gain/1, Switch1/1
  Gain/1 -> Switch1/3
  Target Time Early Swing/1 -> Switch2/1
  Target Time Late Swing/1 -> Switch2/3
  " Timer Phase 1"/1(Out) -> Switch16/1
  " Timer Phase 2"/1(Out) -> Compare To Constant/1, Switch16/3
  Mux5/1 -> State Hip Roll/1, State Ankle/1, State Knee/1, State Hip/1, To Workspace3/1
  Mux/1 -> To Workspace1/1
  Minimal jerk Hip Pitch1/1(jerk) -> Mux/1, Integrator/1
  Minimal jerk Hip Pitch2/1(jerk) -> Mux/2, Integrator3/1
  Minimal jerk Hip Pitch3/1(jerk) -> Integrator1/1
  Minimal jerk Hip Pitch4/1(jerk) -> Mux/4, Integrator2/1
  Saturation1/1 -> Product/1
  Compare To Constant/1 -> Switch/2
  Constant/1 -> Switch/3
  Constant1/1 -> Switch/1
  Switch/1 -> Product/2
  Product/1 -> "Desired Acceleration "/1
  Constant2/1 -> Mux/3

== system nmsRR/Supraspinal Level/Subsystem/Compute Target States ==
  note: Target Joint States: Target joint angles, angle velocities and angle acceleration are defined here. For knee and ankle, values are constant. For hip pitch and hip roll, values are computed using the Balance Control mechanism from [Yin et. al. 2007].
      | Low pass filters are added here to compensate for abrupt changes in target angles at transitions between early and late swing.
  Left/Right : Inport
  Early/Late Swing : Inport  Port=2
  Balance Control lateral : Subsystem
  Balance Control saggital : Subsystem
  Constant : Constant  Value=1.4
  Constant1 : Constant  Value=100
  Constant{5..6,11,20..22} (6 alike) : Constant  Value=0
  Constant13 : Constant  Value=pi
  Constant23 : Constant  Value=20
  Constant24 : Constant  Value=20
  Gain3 : Gain  Gain=-1
  Minus1 : Sum
  Minus8 : Sum  Inputs=+++
  Mux{2..3,5..6} (4 alike) : Mux  Inputs=3
  Switch19 : Switch  Criteria=u2 > Threshold
  Transfer Fcn (with initial outputs) : simulink_extras/Additional Linear/Transfer Fcn (with initial outputs)  N=[1]  D="[0.1  1]"  Y0=init_angle_sag  U0=init_angle_sag
  Transfer Fcn (with initial outputs)1 : simulink_extras/Additional Linear/Transfer Fcn (with initial outputs)  N=[1]  D="[0.1  1]"  Y0=init_angle_lat  U0=init_angle_lat
  Hip Pitch Target : Outport
  Knee Target : Outport  Port=2
  Ankle Target : Outport  Port=3
  Hip Roll Target : Outport  Port=4
  wires:
  Constant22/1 -> Mux5/3
  [TrunkRot_sag] -> Minus8/3
  Minus8/1 -> Transfer Fcn (with initial outputs)/1
  Constant20/1 -> Mux3/3
  Constant23/1 -> Switch19/1
  Transfer Fcn (with initial outputs)1/1 -> Mux2/1
  Mux3/1 -> Hip Pitch Target/1
  Left/Right/1 -> Balance Control lateral/1(Left/Right), Balance Control saggital/1(Left/Right)
  Minus1/1 -> Transfer Fcn (with initial outputs)1/1
  Early/Late Swing/1 -> Switch19/2
  Constant/1 -> Mux6/1
  Mux2/1 -> Hip Roll Target/1
  Gain3/1 -> Minus8/1
  Constant1/1 -> Switch19/3
  Mux6/1 -> Ankle Target/1
  Constant21/1 -> Mux5/2
  Constant6/1 -> Mux2/3
  Constant5/1 -> Mux2/2
  Balance Control lateral/1(theta_Hip_swing_target) -> Minus1/1
  Balance Control saggital/1(theta_Hip_swing_target) -> Gain3/1
  Mux5/1 -> Knee Target/1
  Constant11/1 -> Mux3/2
  Constant13/1 -> Minus8/2
  [TrunkRot_lat] -> Minus1/2
  Constant24/1 -> Mux6/2
  Switch19/1 -> Mux6/3
  [swk] -> Mux5/1
  Transfer Fcn (with initial outputs)/1 -> Mux3/1

== system nmsRR/Supraspinal Level/Subsystem/Inverse Dynamics ==
  Desired Acceleration : Inport
  Inverse Dynamics : Subsystem
  Sensor Data from Body Layer : Subsystem
  Desired Torques : Outport
  wires:
  Inverse Dynamics/1(" Desired Torques") -> Desired Torques/1
  Desired Acceleration/1 -> Inverse Dynamics/7(Desired Acceleration [rad/s^2])
  Sensor Data from Body Layer/1(" Rotation Trunk [rad]") -> Inverse Dynamics/1(Rotation Trunk [rad])
  Sensor Data from Body Layer/2(Joint Angle Velocities [rad/s]) -> Inverse Dynamics/2(Joint Angle Velocities [rad/s])
  Sensor Data from Body Layer/3(Joint Angles [rad]) -> Inverse Dynamics/3(Joint Angles [rad])
  Sensor Data from Body Layer/4(Rotation Velocity Trunk [rad/s]) -> Inverse Dynamics/4(Rotation Velocity Trunk [rad/s])
  Sensor Data from Body Layer/5(Trunk Position [m]) -> Inverse Dynamics/5(Trunk Position [m])
  Sensor Data from Body Layer/6(Trunk Velocity [m/s]) -> Inverse Dynamics/6(Trunk Velocity [m/s])

== system nmsRR/Supraspinal Level/Subsystem/Inversion of Muscle Model ==
  note: Inversion of Muscle Model: This block implements the inversion of the Hill-type muscle model.
  Desired Forces : Inport
  Demux : Demux  Outputs=22
  Divide1 : Product  Inputs=*/
  Divide11 : Product  Inputs=*/
  Fmax1 : Gain  Gain=1./mParams.muscles.FmaxVec  SaturateOnIntegerOverflow=on  OutDataTypeStr=Inherit: Same as input  ParamDataTypeStr=Inherit: Same as input
  Fmax4 : Gain  Gain=1./mParams.muscles.FmaxVec  SaturateOnIntegerOverflow=on  OutDataTypeStr=Inherit: Same as input  ParamDataTypeStr=Inherit: Same as input
  Multiply2 : Product
  Multiply6 : Product
  Mux : Mux  Inputs=11
  Mux1 : Mux  Inputs=11
  Saturation{1..3,5} (4 alike) : Saturate  UpperLimit=inf  LowerLimit=0.00005  ZeroCross=off
  Desired Activation Left : Outport
  Desired Activation Right : Outport  Port=2
  wires:
  Saturation1/1 -> Multiply6/1
  Demux/3 -> Mux/3
  Demux/9 -> Mux/9
  Demux/21 -> Mux1/10
  Demux/6 -> Mux/6
  Multiply6/1 -> Divide11/2
  Demux/11 -> Mux/11
  Demux/2 -> Mux/2
  Demux/7 -> Mux/7
  Mux/1 -> Fmax1/1
  Demux/19 -> Mux1/8
  Mux1/1 -> Fmax4/1
  [fl_R] -> Saturation2/1
  Desired Forces/1 -> Demux/1
  Demux/20 -> Mux1/9
  Demux/4 -> Mux/4
  [fl_L] -> Saturation5/1
  Demux/8 -> Mux/8
  Divide1/1 -> Desired Activation Left/1
  Demux/1 -> Mux/1
  Demux/14 -> Mux1/3
  Demux/12 -> Mux1/1
  Fmax4/1 -> Divide11/1
  Saturation3/1 -> Multiply2/1
  [fv_R] -> Saturation1/1
  Demux/5 -> Mux/5
  Saturation5/1 -> Multiply2/2
  Demux/15 -> Mux1/4
  [fv_L] -> Saturation3/1
  Demux/18 -> Mux1/7
  Multiply2/1 -> Divide1/2
  Saturation2/1 -> Multiply6/2
  Demux/10 -> Mux/10
  Demux/16 -> Mux1/5
  Demux/22 -> Mux1/11
  Fmax1/1 -> Divide1/1
  Demux/13 -> Mux1/2
  Divide11/1 -> Desired Activation Right/1
  Demux/17 -> Mux1/6

== system nmsRR/Supraspinal Level/Subsystem/Stretch Reflex Inversion ==
  note: Inversion of Stretch: This block implements the inversion of the tonic stretch reflex.
  Desired Activation Left : Inport
  Desired Activation Right : Inport  Port=2
  Gain1 : Gain  Gain=-1/mParams.muscles.K
  Gain12 : Gain  Gain=-1/mParams.muscles.K
  Sum14 : Sum  Inputs=|++
  Sum2 : Sum  Inputs=|++
  Descending Command Left : Outport
  Descending Command Right : Outport  Port=2
  wires:
  Desired Activation Right/1 -> Gain12/1
  Sum14/1 -> Descending Command Right/1
  Desired Activation Left/1 -> Gain1/1
  Sum2/1 -> Descending Command Left/1
  [RLceVec] -> Sum14/2
  Gain12/1 -> Sum14/1
  Gain1/1 -> Sum2/1
  [LLceVec] -> Sum2/2

== system nmsRR/Supraspinal Level/Subsystem/torques --> forces ==
  note: Desired Forces: Desired Forces are computed by an iterative approach. The pseudoinverse-method is used to compute forces that generate the desired force profiles. This forces, however, can potentially be negative unlike real muscle forces. Therefore, torques that these negative forces would produce are computed. The resulting torques are again transformed into forces that have a smaller negative component now. This procedure is repeated 6 times.
  note: Moment Arm Matrix (C) and its Inverse (C_transpose)
  Desired Torque : Inport
  Add13 : Sum  Inputs=++++++
  F from T2 : Subsystem
  Gain : Gain  Gain=-1
  Moment Arm Matrix : Subsystem
  Pseudoinverse : dspinverses/Pseudoinverse  wanterr=off  SimulateUsing=Code generation
      settings: SourceProductBaseCode=DS
  Separate Force : Subsystem
  Subsystem1 : Subsystem
  Subsystem12 : Subsystem
  Subsystem2 : Subsystem
  Subsystem3 : Subsystem
  Subsystem4 : Subsystem
  Terminator : Terminator
  Transpose : Math  Operator=transpose  SaturateOnIntegerOverflow=on
  Desired Force : Outport
  tag scope: C=global, C_transpose=global
  wires:
  Desired Torque/1 -> F from T2/1(Desired Torques)
  F from T2/1(Desired Forces) -> Separate Force/1(Force)
  Add13/1 -> Desired Force/1
  Separate Force/1(Positive) -> Add13/1
  Subsystem1/1(Positive Part) -> Add13/6
  Subsystem4/1(Positive Part) -> Add13/5
  Subsystem4/2(Negative Part) -> Subsystem1/1(Force)
  Subsystem3/1(Positive Part) -> Add13/4
  Subsystem3/2(Negative Part) -> Subsystem4/1(Force)
  Subsystem2/1(Positive Part) -> Add13/3
  Subsystem2/2(Negative Part) -> Subsystem3/1(Force)
  Separate Force/2(Negative) -> Subsystem12/1(Force)
  Subsystem12/1(Positive Part) -> Add13/2
  Subsystem12/2(Negative Part) -> Subsystem2/1(Force)
  Subsystem1/2(Negative Part) -> Terminator/1
  Transpose/1 -> Pseudoinverse/1
  [Llegq] -> Moment Arm Matrix/1(Lleg)
  Pseudoinverse/1 -> [C_transpose]
  Moment Arm Matrix/1(Moment Arm Matrix) -> Gain/1
  [Rlegq] -> Moment Arm Matrix/2(Rleg)
  Gain/1 -> [C], Transpose/1

== system nmsRR/Body and Contact Model/L Leg/Foot/  XYZ Sensor Ball left ==
  note: Simplified IMU Model
  Frame Sensor : sm_lib/Frames and Transforms/Transform Sensor  MeasurementFrame=World  SenseAngle=off  SenseAxis=off  SenseAngle1=off  SenseAngle2=off  SenseAngle3=off  SenseQ=off  SenseR=off  SenseOmegaX=off  SenseOmegaY=off  SenseOmegaZ=off  SenseOmega1=off  SenseOmega2=off  SenseOmega3=off  SenseQDot=off  SenseRDot=off  SenseAlphaX=off  SenseAlphaY=off  SenseAlphaZ=off  SenseAlpha1=off  SenseAlpha2=off  SenseAlpha3=off  SenseQDDot=off  SenseRDDot=off  SenseX=on  SenseY=on  SenseZ=on  SenseRad=off  SenseAzim=off  SenseDist=off  SenseInc=off  SenseXDot=on  SenseYDot=on  SenseZDot=on  SenseRadDot=off  SenseAzimDot=off  SenseDistDot=off  SenseIncDot=off  SenseXDDot=off  SenseYDDot=off  SenseZDDot=off  SenseRadDDot=off  SenseAzimDDot=off  SenseDistDDot=off  SenseIncDDot=off
  Mux3 : Mux  Inputs=3
  Mux4 : Mux  Inputs=3
  PS-Simulink Converter : nesl_utility/PS-Simulink Converter  PhysicalDomain=network_engine_domain  SubClassName=ps_output  LeftPortType=input  RightPortType=output  PseudoPeriodic=off  Frequencies=[]  Unit=m  AffineConversion=off
      settings: SourceProductBaseCode=PW,SS
  PS-Simulink Converter1 : nesl_utility/PS-Simulink Converter  PhysicalDomain=network_engine_domain  SubClassName=ps_output  LeftPortType=input  RightPortType=output  PseudoPeriodic=off  Frequencies=[]  Unit=m  AffineConversion=off
      settings: SourceProductBaseCode=PW,SS
  PS-Simulink Converter2 : nesl_utility/PS-Simulink Converter  PhysicalDomain=network_engine_domain  SubClassName=ps_output  LeftPortType=input  RightPortType=output  PseudoPeriodic=off  Frequencies=[]  Unit=m/s  AffineConversion=off
      settings: SourceProductBaseCode=PW,SS
  PS-Simulink Converter3 : nesl_utility/PS-Simulink Converter  PhysicalDomain=network_engine_domain  SubClassName=ps_output  LeftPortType=input  RightPortType=output  PseudoPeriodic=off  Frequencies=[]  Unit=m/s  AffineConversion=off
      settings: SourceProductBaseCode=PW,SS
  PS-Simulink Converter4 : nesl_utility/PS-Simulink Converter  PhysicalDomain=network_engine_domain  SubClassName=ps_output  LeftPortType=input  RightPortType=output  PseudoPeriodic=off  Frequencies=[]  Unit=m  AffineConversion=off
      settings: SourceProductBaseCode=PW,SS
  PS-Simulink Converter5 : nesl_utility/PS-Simulink Converter  PhysicalDomain=network_engine_domain  SubClassName=ps_output  LeftPortType=input  RightPortType=output  PseudoPeriodic=off  Frequencies=[]  Unit=m/s  AffineConversion=off
      settings: SourceProductBaseCode=PW,SS
  World Frame : sm_lib/Frames and Transforms/World Frame
  frame : PMIOPort  Side=Left
  p_bLH [m x3] : Outport  VectorParamsAs1DForOutWhenUnconnected=off
  v_bLH [m/s x3] : Outport  Port=2  VectorParamsAs1DForOutWhenUnconnected=off
  wires:
  PS-Simulink Converter4/1 -> Mux3/3
  PS-Simulink Converter3/1 -> Mux4/2
  PS-Simulink Converter5/1 -> Mux4/3
  PS-Simulink Converter/1 -> Mux3/1
  Mux3/1 -> p_bLH [m x3]/1
  Mux4/1 -> v_bLH [m/s x3]/1
  PS-Simulink Converter2/1 -> Mux4/1
  PS-Simulink Converter1/1 -> Mux3/2
  connections:
  Frame Sensor/RConn1 -- frame/RConn1
  World Frame/RConn1 -- Frame Sensor/LConn1
  Frame Sensor/RConn2 -- PS-Simulink Converter/LConn1
  Frame Sensor/RConn3 -- PS-Simulink Converter1/LConn1
  Frame Sensor/RConn4 -- PS-Simulink Converter4/LConn1
  Frame Sensor/RConn5 -- PS-Simulink Converter2/LConn1
  Frame Sensor/RConn6 -- PS-Simulink Converter3/LConn1
  Frame Sensor/RConn7 -- PS-Simulink Converter5/LConn1

== system nmsRR/Body and Contact Model/Push in x-direction/ Timer Phase 1/Resettable Subsystem ==
  In1 : Inport
  Enable : EnablePort  ZeroCross=off
  Out1 : Outport
  wires:
  In1/1 -> Out1/1

== system nmsRR/Body and Contact Model/Push in y-direction/ Timer Phase 1/Resettable Subsystem ==
  In1 : Inport
  Enable : EnablePort  ZeroCross=off
  Out1 : Outport
  wires:
  In1/1 -> Out1/1

== system nmsRR/Body and Contact Model/R Leg/Foot1/  XYZ Sensor  ==
  note: Simplified IMU Model
  Frame Sensor : sm_lib/Frames and Transforms/Transform Sensor  MeasurementFrame=World  SenseAngle=off  SenseAxis=off  SenseAngle1=off  SenseAngle2=off  SenseAngle3=off  SenseQ=off  SenseR=off  SenseOmegaX=off  SenseOmegaY=off  SenseOmegaZ=off  SenseOmega1=off  SenseOmega2=off  SenseOmega3=off  SenseQDot=off  SenseRDot=off  SenseAlphaX=off  SenseAlphaY=off  SenseAlphaZ=off  SenseAlpha1=off  SenseAlpha2=off  SenseAlpha3=off  SenseQDDot=off  SenseRDDot=off  SenseX=on  SenseY=on  SenseZ=on  SenseRad=off  SenseAzim=off  SenseDist=off  SenseInc=off  SenseXDot=on  SenseYDot=on  SenseZDot=on  SenseRadDot=off  SenseAzimDot=off  SenseDistDot=off  SenseIncDot=off  SenseXDDot=off  SenseYDDot=off  SenseZDDot=off  SenseRadDDot=off  SenseAzimDDot=off  SenseDistDDot=off  SenseIncDDot=off
  Mux3 : Mux  Inputs=3
  Mux4 : Mux  Inputs=3
  PS-Simulink Converter : nesl_utility/PS-Simulink Converter  PhysicalDomain=network_engine_domain  SubClassName=ps_output  LeftPortType=input  RightPortType=output  PseudoPeriodic=off  Frequencies=[]  Unit=m  AffineConversion=off
      settings: SourceProductBaseCode=PW,SS
  PS-Simulink Converter1 : nesl_utility/PS-Simulink Converter  PhysicalDomain=network_engine_domain  SubClassName=ps_output  LeftPortType=input  RightPortType=output  PseudoPeriodic=off  Frequencies=[]  Unit=m  AffineConversion=off
      settings: SourceProductBaseCode=PW,SS
  PS-Simulink Converter2 : nesl_utility/PS-Simulink Converter  PhysicalDomain=network_engine_domain  SubClassName=ps_output  LeftPortType=input  RightPortType=output  PseudoPeriodic=off  Frequencies=[]  Unit=m/s  AffineConversion=off
      settings: SourceProductBaseCode=PW,SS
  PS-Simulink Converter3 : nesl_utility/PS-Simulink Converter  PhysicalDomain=network_engine_domain  SubClassName=ps_output  LeftPortType=input  RightPortType=output  PseudoPeriodic=off  Frequencies=[]  Unit=m/s  AffineConversion=off
      settings: SourceProductBaseCode=PW,SS
  PS-Simulink Converter4 : nesl_utility/PS-Simulink Converter  PhysicalDomain=network_engine_domain  SubClassName=ps_output  LeftPortType=input  RightPortType=output  PseudoPeriodic=off  Frequencies=[]  Unit=m  AffineConversion=off
      settings: SourceProductBaseCode=PW,SS
  PS-Simulink Converter5 : nesl_utility/PS-Simulink Converter  PhysicalDomain=network_engine_domain  SubClassName=ps_output  LeftPortType=input  RightPortType=output  PseudoPeriodic=off  Frequencies=[]  Unit=m/s  AffineConversion=off
      settings: SourceProductBaseCode=PW,SS
  World Frame : sm_lib/Frames and Transforms/World Frame
  frame : PMIOPort  Side=Left
  p_bLH [m x3] : Outport  VectorParamsAs1DForOutWhenUnconnected=off
  v_bLH [m/s x3] : Outport  Port=2  VectorParamsAs1DForOutWhenUnconnected=off
  wires:
  PS-Simulink Converter4/1 -> Mux3/3
  PS-Simulink Converter3/1 -> Mux4/2
  PS-Simulink Converter5/1 -> Mux4/3
  PS-Simulink Converter/1 -> Mux3/1
  Mux3/1 -> p_bLH [m x3]/1
  Mux4/1 -> v_bLH [m/s x3]/1
  PS-Simulink Converter2/1 -> Mux4/1
  PS-Simulink Converter1/1 -> Mux3/2
  connections:
  Frame Sensor/RConn1 -- frame/RConn1
  World Frame/RConn1 -- Frame Sensor/LConn1
  Frame Sensor/RConn2 -- PS-Simulink Converter/LConn1
  Frame Sensor/RConn3 -- PS-Simulink Converter1/LConn1
  Frame Sensor/RConn4 -- PS-Simulink Converter4/LConn1
  Frame Sensor/RConn5 -- PS-Simulink Converter2/LConn1
  Frame Sensor/RConn6 -- PS-Simulink Converter3/LConn1
  Frame Sensor/RConn7 -- PS-Simulink Converter5/LConn1

== system nmsRR/Body and Contact Model/R Leg/Foot1/  XYZ Sensor Ball left ==
  note: Simplified IMU Model
  Frame Sensor : sm_lib/Frames and Transforms/Transform Sensor  MeasurementFrame=World  SenseAngle=off  SenseAxis=off  SenseAngle1=off  SenseAngle2=off  SenseAngle3=off  SenseQ=off  SenseR=off  SenseOmegaX=off  SenseOmegaY=off  SenseOmegaZ=off  SenseOmega1=off  SenseOmega2=off  SenseOmega3=off  SenseQDot=off  SenseRDot=off  SenseAlphaX=off  SenseAlphaY=off  SenseAlphaZ=off  SenseAlpha1=off  SenseAlpha2=off  SenseAlpha3=off  SenseQDDot=off  SenseRDDot=off  SenseX=on  SenseY=on  SenseZ=on  SenseRad=off  SenseAzim=off  SenseDist=off  SenseInc=off  SenseXDot=on  SenseYDot=on  SenseZDot=on  SenseRadDot=off  SenseAzimDot=off  SenseDistDot=off  SenseIncDot=off  SenseXDDot=off  SenseYDDot=off  SenseZDDot=off  SenseRadDDot=off  SenseAzimDDot=off  SenseDistDDot=off  SenseIncDDot=off
  Mux3 : Mux  Inputs=3
  Mux4 : Mux  Inputs=3
  PS-Simulink Converter : nesl_utility/PS-Simulink Converter  PhysicalDomain=network_engine_domain  SubClassName=ps_output  LeftPortType=input  RightPortType=output  PseudoPeriodic=off  Frequencies=[]  Unit=m  AffineConversion=off
      settings: SourceProductBaseCode=PW,SS
  PS-Simulink Converter1 : nesl_utility/PS-Simulink Converter  PhysicalDomain=network_engine_domain  SubClassName=ps_output  LeftPortType=input  RightPortType=output  PseudoPeriodic=off  Frequencies=[]  Unit=m  AffineConversion=off
      settings: SourceProductBaseCode=PW,SS
  PS-Simulink Converter2 : nesl_utility/PS-Simulink Converter  PhysicalDomain=network_engine_domain  SubClassName=ps_output  LeftPortType=input  RightPortType=output  PseudoPeriodic=off  Frequencies=[]  Unit=m/s  AffineConversion=off
      settings: SourceProductBaseCode=PW,SS
  PS-Simulink Converter3 : nesl_utility/PS-Simulink Converter  PhysicalDomain=network_engine_domain  SubClassName=ps_output  LeftPortType=input  RightPortType=output  PseudoPeriodic=off  Frequencies=[]  Unit=m/s  AffineConversion=off
      settings: SourceProductBaseCode=PW,SS
  PS-Simulink Converter4 : nesl_utility/PS-Simulink Converter  PhysicalDomain=network_engine_domain  SubClassName=ps_output  LeftPortType=input  RightPortType=output  PseudoPeriodic=off  Frequencies=[]  Unit=m  AffineConversion=off
      settings: SourceProductBaseCode=PW,SS
  PS-Simulink Converter5 : nesl_utility/PS-Simulink Converter  PhysicalDomain=network_engine_domain  SubClassName=ps_output  LeftPortType=input  RightPortType=output  PseudoPeriodic=off  Frequencies=[]  Unit=m/s  AffineConversion=off
      settings: SourceProductBaseCode=PW,SS
  World Frame : sm_lib/Frames and Transforms/World Frame
  frame : PMIOPort  Side=Left
  p_bLH [m x3] : Outport  VectorParamsAs1DForOutWhenUnconnected=off
  v_bLH [m/s x3] : Outport  Port=2  VectorParamsAs1DForOutWhenUnconnected=off
  wires:
  PS-Simulink Converter4/1 -> Mux3/3
  PS-Simulink Converter3/1 -> Mux4/2
  PS-Simulink Converter5/1 -> Mux4/3
  PS-Simulink Converter/1 -> Mux3/1
  Mux3/1 -> p_bLH [m x3]/1
  Mux4/1 -> v_bLH [m/s x3]/1
  PS-Simulink Converter2/1 -> Mux4/1
  PS-Simulink Converter1/1 -> Mux3/2
  connections:
  Frame Sensor/RConn1 -- frame/RConn1
  World Frame/RConn1 -- Frame Sensor/LConn1
  Frame Sensor/RConn2 -- PS-Simulink Converter/LConn1
  Frame Sensor/RConn3 -- PS-Simulink Converter1/LConn1
  Frame Sensor/RConn4 -- PS-Simulink Converter4/LConn1
  Frame Sensor/RConn5 -- PS-Simulink Converter2/LConn1
  Frame Sensor/RConn6 -- PS-Simulink Converter3/LConn1
  Frame Sensor/RConn7 -- PS-Simulink Converter5/LConn1

== system nmsRR/Body and Contact Model/Vestibular System/Align Axis/Compute Lateral Rotation ==
  Hip Left : Inport
  Hip Right : Inport  Port=2
  Constant : Constant  Value=[0 0 1]
  Constant1 : Constant
  Constant2 : Constant  Value=-1
  Dot Product : DotProduct  InputSameDT=on  OutDataTypeStr=Inherit: Inherit via internal rule
  Minus : Sum  Inputs=+-
  Product : Product
  Selector : Selector  InputPortWidth=3  IndexOptions=Index vector (dialog)  Indices=[2]  OutputSizes=1
  Switch : Switch  Criteria=u2 > Threshold
  Trigonometric Function : Trigonometry  Operator=acos
  normalize : Subsystem
  Lateral Rotation : Outport
  wires:
  Hip Right/1 -> Minus/1
  Selector/1 -> Switch/2
  Product/1 -> Lateral Rotation/1
  Constant2/1 -> Switch/1
  Constant/1 -> Dot Product/1
  Constant1/1 -> Switch/3
  Switch/1 -> Product/1
  Trigonometric Function/1 -> Product/2
  Minus/1 -> normalize/1(vector)
  normalize/1(norm) -> Dot Product/2, Selector/1
  Dot Product/1 -> Trigonometric Function/1
  Hip Left/1 -> Minus/2
